simulink model "phdMain"  (R2023b)
settings: Solver=ode4  StartTime=0.0  StopTime=t.Data(end)  FixedStep=1e-3  RelTol=1e-3
undefined symbols (not defined in the file): A_bar, AEFF, B_E, C_bar, C_T, Cd_neg, Cd_pos, DiscIntNeverNeededParam, Gamma, H, k, K, L_gain, L_STROKE, M, m3PsToLpm, P_return_Pa, P_supply_Pa, PA_Pa, PaToBar, PB_Pa, Q, R, RHO, Ts, V01, V02, V_DEAD, v_mPs, W, xc_dot, xc_m
libraries: simulink x1
(part 1 of 3)
settings Model: PauseTimes=22  Creator=snr  LastModifiedBy=snr
settings DataIOCC: OutputOption=AdditionalOutputTimes  OutputTimes=1
settings OptimizationCC: BlockReduction=off  ConditionallyExecuteInputs=off

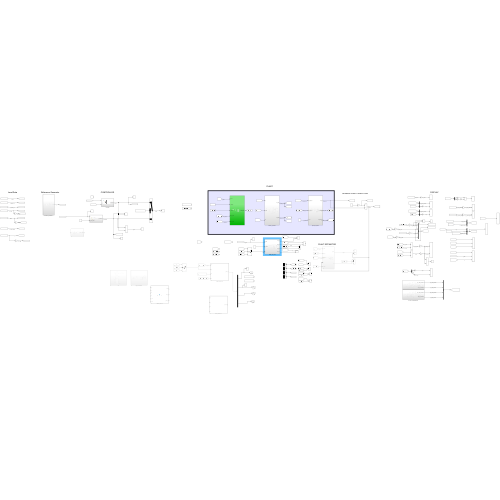
[thumbnail: Simulink's stored preview of the top-level diagram]
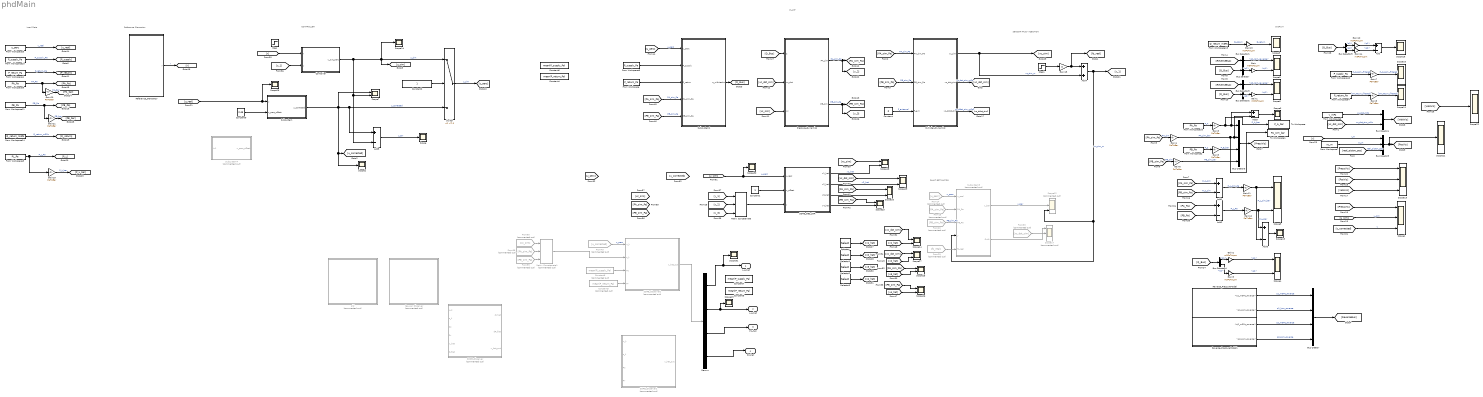
== system phdMain ==
  note: Load Data
  note: PLANT
  note: CONTROLLER
  note: DISPLAY
  note: Reference Generator
  note: SENSOR FAULT INJECTION
  note: FAULT ESTIMATOR
  Add{,1..3,5..6} (6 alike) : Sum  Inputs=+-
  Add4 : Sum
  Bus Selector : BusSelector  OutputSignals=q1
  Bus Selector1 : BusSelector  OutputSignals=q1_lpm_reverse
  Bus Selector2 : BusSelector  OutputSignals=q2
  Bus Selector3 : BusSelector  OutputSignals=q2_lpm_reverse
  Bus Selector4 : BusSelector  OutputSignals=q1,q2
  Bus Selector5 : BusSelector  OutputSignals=q1,q2
  Bus Creator : BusCreator  Inputs=4
  Bus Creator3 : BusCreator  Inputs=4
  Bus Creator4 : BusCreator  Inputs=2
  Bus Creator5 : BusCreator  Inputs=3
  Constant : Constant  Value=0
  Constant1 : Constant
  Constant2 : Constant  OutDataTypeStr=boolean
  Constant3 : Constant  Commented=on  Value=mean(P_return_Pa)
  Constant4 : Constant  Value=mean(P_return_Pa)
  Constant5 : Constant  Value=mean(P_return_Pa)
  Constant6 : Constant  Value=mean(P_supply_Pa)
  Constant7 : Constant  Value=mean(P_supply_Pa)
  Constant8 : Constant  Commented=on  Value=mean(P_supply_Pa)
  Constant9 : Constant  Value=2.45
  Controller : Subsystem
  Cylinder_Dynamics : Subsystem
  Demux : Demux
  From Workspace : FromWorkspace  VariableName=P_return_Pa
  From Workspace1 : FromWorkspace  VariableName=P_return_Pa
  From Workspace10 : FromWorkspace  VariableName=P_supply_Pa
  From Workspace11 : FromWorkspace  VariableName=PB_Pa
  From Workspace12 : FromWorkspace  VariableName=P_supply_Pa
  From Workspace14 : FromWorkspace  VariableName=Q_return_m3Ps
  From Workspace15 : FromWorkspace  VariableName=Q_return_m3Ps
  From Workspace2 : FromWorkspace  VariableName=PB_Pa
  From Workspace20 : FromWorkspace  VariableName=PA_Pa
  From Workspace3 : FromWorkspace  VariableName=u_perc
  From Workspace4 : FromWorkspace  VariableName=P_return_Pa
  From Workspace5 : FromWorkspace  VariableName=PL_Pa
  From Workspace6 : FromWorkspace  VariableName=v_mPs
  From Workspace7 : FromWorkspace  VariableName=xc_m
  From Workspace8 : FromWorkspace  VariableName=P_supply_Pa
  From Workspace9 : FromWorkspace  VariableName=PA_Pa
  From14 : From  Commented=on  GotoTag=u_perc
  From15 : From  Commented=on  GotoTag=PA_sim_Pa
  From20 : From  Commented=on  GotoTag=PB_sim_Pa
  From29 : From  Commented=on  GotoTag=fs_real
  From33 : From  Commented=on  GotoTag=xc_dot_sim
  From43 : From  Commented=on  GotoTag=u_corrected
  From58 : From  Commented=on  GotoTag=PA_sim_Pa
  From59 : From  Commented=on  GotoTag=PB_sim_Pa
  From60 : From  Commented=on  GotoTag=xc_sim
  Gain{,1..2,9..10,13..14} (7 alike) : Gain  Gain=m3PsToLpm
  Gain{3..8,11..12,19..21} (11 alike) : Gain  Gain=PaToBar
  Gain15 : Gain  Gain=0
  Matrix Concatenate : Concatenate  NumInputs=3  Mode=Multidimensional array
  Matrix Concatenate1 : Concatenate  Commented=on  NumInputs=3  Mode=Multidimensional array
  Nguyen Observer : Subsystem  Commented=on
  Pressure_Dynamics : Subsystem
  Reference_Generator : Subsystem
  Reverse_PressureModel : Subsystem
  Reverse_PressureModel1 : Subsystem
  SDRE_OBS_SNR : Subsystem
  SDRE_Observer : MATLAB Function  Commented=on  InitFcn=% x_hat Integrator IC x0_obs = [0; 0; 0; 0]; % 4×1 % P Integrator IC P0 = diag([1e-5, 1e-3, 2e3, 2e3]); % 4×4 P0_flat = P0(:); % 16×1 ← bu kullanılacak  TreatAsAtomicUnit=on
  SDRE_Observer1 : MATLAB Function  Commented=on  TreatAsAtomicUnit=on
  SDRE_Observer2 : MATLAB Function  Commented=on  TreatAsAtomicUnit=on
  Scope{,2..3,8,10..11,14..16,19,21..22,28,30..31} (15 alike) : Scope
  Scope1 : Scope  NumInputPorts=3
  Scope12 : Scope  Commented=on  NumInputPorts=3
  Scope13 : Scope  NumInputPorts=3
  Scope17 : Scope  Commented=on  NumInputPorts=3
  Scope{4..7,9,18,20,23..27,29} (13 alike) : Scope  NumInputPorts=2
  Selector{,1..3} (4 alike) : Selector  InputPortWidth=4  IndexOptions=Index vector (dialog)  Indices=1  OutputSizes=1
  Step : Step  After=10e-3  SampleTime=0
  Step1 : Step  After=5e-3  SampleTime=0
  Subsystem : Subsystem
  Subsystem1 : Subsystem
  Subsystem3 : Subsystem  Commented=on
  Subsystem4 : Subsystem  Commented=on
  Switch : Switch  Criteria=u2 ~= 0  SaturateOnIntegerOverflow=off  InputSameDT=off
  To Workspace : ToWorkspace  VariableName=P_A_bar  SaveFormat=Timeseries  SampleTime=-1
  To Workspace1 : ToWorkspace  VariableName=PA_sim_bar  SaveFormat=Timeseries  SampleTime=-1
  old : Subsystem  Commented=on
  x_c_hat : Outport
  v_c_hat : Outport  Port=2
  P1_hat : Outport  Port=3
  P2_hat : Outport  Port=4
  wires:
  Constant/1 -> Cylinder_Dynamics/3(F_ext)  "F_external"
  Cylinder_Dynamics/2(xc_dot_sim) -> [xc_dot_sim]  "xc_dot_sim_mPs"
  From Workspace7/1 -> Bus Creator5/2  "xc_m"
  [real_piston_pos] -> Bus Creator5/3  "real_piston_pos"
  [xc_dot_sim] -> Bus Creator4/2  "xc_dot_sim_mPs"
  From Workspace6/1 -> Bus Creator4/1  "xc_dot_mPs"
  Pressure_Dynamics/1(PA_sim) -> [y_2], [PA_sim_Pa]  "PA_sim_Pa"
  [PA_sim_Pa] -> Cylinder_Dynamics/1(PA_sim_Pa)  "PA_sim_Pa"
  Pressure_Dynamics/2(PB_sim) -> [y_3], [PB_sim_Pa]  "PB_sim_Pa"
  [PB_sim_Pa] -> Cylinder_Dynamics/2(PB_sim_Pa)  "PB_sim_Pa"
  From Workspace20/1 -> Gain3/1  "P_A"
  [PA_sim_Pa] -> Gain4/1  "PA_sim"
  [PB_sim_Pa] -> Gain6/1  "PB_sim"
  From Workspace2/1 -> Gain5/1  "P_2"
  [Q_Bus] -> Bus Selector/1
  [ReverseBus] -> Bus Selector1/1
  Bus Selector/1 -> Gain/1  "<q1>"
  Bus Selector1/1 -> Scope5/1  "<q1_lpm_reverse>"
  Gain/1 -> Scope5/2  "<q1>"
  Gain1/1 -> Scope6/2  "<q2>"
  Bus Selector3/1 -> Scope6/1  "<q2_lpm_reverse>"
  Bus Selector2/1 -> Gain1/1  "<q2>"
  [ReverseBus] -> Bus Selector3/1
  [Q_Bus] -> Bus Selector2/1
  [xc_sim] -> Pressure_Dynamics/3(xc)
  [xc_dot_sim] -> Pressure_Dynamics/2(xc_dot)
  [PA_sim_Pa] -> Add1/1  "P_1_sim"
  [PB_sim_Pa] -> Add1/2  "P_2_sim"
  Switch/1 -> [u_perc]  "u_sim"
  Add1/1 -> Gain11/1  "P_L_sim_Pa"
  Add2/1 -> Gain12/1  "P_L_Pa"
  Gain3/1 -> To Workspace/1, Add3/1, Bus Creator3/1  "P_A_bar"
  Gain4/1 -> To Workspace1/1, Add3/2, Bus Creator3/2  "PA_sim_bar"
  Gain6/1 -> Bus Creator3/4  "PB_sim_bar"
  Gain5/1 -> Bus Creator3/3  "P_B_bar"
  From Workspace12/1 -> Gain7/1  "P_supply_filtered"
  Gain7/1 -> Scope10/1  "P_supply_filtered"
  Gain8/1 -> Scope11/1  "[t,P_return_filtered]"
  From Workspace4/1 -> Gain8/1  "[t,P_return_filtered]"
  Bus Creator3/1 -> [PressVis]
  [PressVis] -> Scope13/1
  Bus Creator4/1 -> [VeloVis]
  Bus Creator5/1 -> Scope21/1, [PosVis]
  [PressVis] -> Scope1/1
  Gain11/1 -> Add6/2, Scope9/1  "P_L_sim_bar"
  Gain12/1 -> Add6/1, Scope9/2  "P_L_bar"
  Add3/1 -> Scope3/1
  Bus Selector4/1 -> Gain2/1  "<q1>"
  [Q_Bus] -> Bus Selector4/1
  Gain2/1 -> Scope4/1  "<q1>"
  Bus Selector4/2 -> Gain9/1  "<q2>"
  Gain9/1 -> Scope4/2  "<q2>"
  From Workspace15/1 -> Gain13/1  "Q_return"
  Gain13/1 -> Scope8/1  "Q_return"
  [u_corrected] -> Scope1/3  "u"
  Gain10/1 -> Add/1  "<q1>"
  Bus Selector5/1 -> Gain10/1  "<q1>"
  [Q_Bus] -> Bus Selector5/1
  Bus Selector5/2 -> Gain14/1  "<q2>"
  Gain14/1 -> Add/2  "<q2>"
  Add/1 -> Scope16/1
  Constant2/1 -> Switch/2
  Controller/1(u_out_perc) -> Scope7/2, Add5/2, Switch/1, [u_sim], Scope14/1  "u_sim"
  Add4/1 -> [y_1], Scope12/3, Subsystem3/4(y)  "xc_sim_m"
  [u_real] -> Scope28/1, Subsystem/1(u)
  Subsystem/1(u_corrected) -> Scope7/1, [u_corrected], Scope2/1, Add5/1, Switch/3  "u_corrected"
  From Workspace3/1 -> [u_real]  "u_real"
  Reverse_PressureModel/2(<q1_lpm_reverse>) -> Bus Creator/2  "q1_lpm_reverse"
  Bus Creator/1 -> [ReverseBus]
  Reverse_PressureModel/1(<q1_m3Ps_reverse>) -> Bus Creator/1  "q1_m3Ps_reverse"
  Reverse_PressureModel1/1(<q2_m3Ps_reverse>) -> Bus Creator/3  "q2_m3Ps_reverse"
  Reverse_PressureModel1/2(<q2_lpm_reverse>) -> Bus Creator/4  "q2_lpm_reverse"
  From Workspace10/1 -> [P_supply]  "P_supply_Pa"
  From Workspace1/1 -> [P_return]  "P_return_Pa"
  From Workspace9/1 -> Gain20/1, [PA_Pa]  "PA_Pa"
  From Workspace11/1 -> Gain21/1, [PB_Pa]  "PB_Pa"
  Cylinder_Dynamics/3(xc_ddot_sim) -> [xc_ddot_sim]  "xc_ddot_sim_mPs2"
  Reference_Generator/1(r) -> [r]  "r"
  From Workspace14/1 -> [Q_return]  "Q_return_m3Ps"
  [PA_Pa] -> Add2/1
  [PB_Pa] -> Add2/2
  From Workspace5/1 -> [P_L], Gain19/1  "P_L_Pa"
  Gain19/1 -> [P_L_bar]  "P_L_bar"
  Gain20/1 -> [PA_bar]  "PA_bar"
  Gain21/1 -> [PB_bar]  "PB_bar"
  Add5/1 -> Scope/1  "u_err"
  Add6/1 -> Scope15/1
  [Q_Bus] -> Pressure_Dynamics/1(q)
  [u_perc] -> Subsystem1/1(u_perc)  "u_perc"
  From Workspace/1 -> Subsystem1/3(P_return)
  [PA_sim_Pa] -> Subsystem1/4(PA_sim_Pa)  "PA_sim_Pa"
  [PB_sim_Pa] -> Subsystem1/5(PB_sim_Pa)  "PB_sim_Pa"
  [VeloVis] -> Scope13/3
  [PosVis] -> Scope13/2
  Subsystem1/1(q_withLeaks) -> [Q_Bus]
  [r] -> Controller/1(r)
  From Workspace8/1 -> Subsystem1/2(P_supply)
  [u_sim] -> Scope1/2  "u_sim"
  [r] -> Bus Creator5/1  "r_m"
  [VeloVis] -> Scope22/1
  From14/1 -> Subsystem3/1(u_real)  "u_perc"
  From15/1 -> Subsystem3/2(PA_Pa)
  From20/1 -> Subsystem3/3(PB_Pa)  "PB_sim_Pa"
  Subsystem3/1(x_bar) -> Scope12/2  "x_bar"
  Cylinder_Dynamics/1(xc_sim) -> Add4/2, [xc_sim]  "xc_sim_m"
  Step1/1 -> Gain15/1
  Gain15/1 -> [fs_real], Add4/1
  From29/1 -> Subsystem3/5(fs_real)
  From33/1 -> Scope17/2
  Subsystem3/2(Out1) -> Scope17/1
  [u_sim] -> Scope30/1, SDRE_OBS_SNR/1(u_real)  "u_perc"
  [y_1] -> Controller/2(y)
  [y_2] -> Matrix Concatenate/2
  [y_1] -> Matrix Concatenate/1
  [y_3] -> Matrix Concatenate/3
  SDRE_OBS_SNR/1(x1_hat) -> Scope18/2  "x1_hat"
  [xc_sim] -> Scope18/1
  SDRE_OBS_SNR/2(x2_hat) -> Scope29/2  "x2_hat"
  [xc_dot_sim] -> Scope29/1
  SDRE_OBS_SNR/3(x3_hat) -> Scope20/2
  [PA_sim_Pa] -> Scope20/1
  SDRE_OBS_SNR/4(x4_hat) -> Scope23/2
  [PB_sim_Pa] -> Scope23/1
  Selector2/1 -> [x3_hat]
  Selector/1 -> [x1_hat]
  Selector1/1 -> [x2_hat]
  Selector3/1 -> [x4_hat]
  [x1_hat] -> Scope24/2
  [xc_dot_sim] -> Scope24/1
  [PA_sim_Pa] -> Scope25/1
  [x3_hat] -> Scope25/2
  [x4_hat] -> Scope26/2
  [PB_sim_Pa] -> Scope26/1
  [xc_dot_sim] -> Scope27/1
  [x2_hat] -> Scope27/2
  Constant1/1 -> SDRE_OBS_SNR/2(u_offset)
  Matrix Concatenate/1 -> SDRE_OBS_SNR/3(y)
  Demux/4 -> P2_hat/1
  Matrix Concatenate1/1 -> SDRE_Observer2/2(z_k)
  Demux/3 -> P1_hat/1
  From59/1 -> Matrix Concatenate1/3
  From60/1 -> Matrix Concatenate1/1
  From58/1 -> Matrix Concatenate1/2
  From43/1 -> SDRE_Observer2/1(u_k)  "u_perc"
  Constant8/1 -> SDRE_Observer2/3(Ps)
  Constant9/1 -> Subsystem/2(u_perc_offset)
  Demux/2 -> Scope19/1, v_c_hat/1
  Constant3/1 -> SDRE_Observer2/4(Pr)
  SDRE_Observer2/1(x_hat_out) -> Demux/1
  Demux/1 -> Scope31/1, x_c_hat/1

== system phdMain/Controller ==
  note: Offset - Yapmaya İhtiyaç yok
  note: Integral Gain
  note: Proportional Gain
  r : Inport  OutDataTypeStr=double
  y : Inport  Port=2  OutDataTypeStr=double
  Add : Sum
  Add1 : Sum  Inputs=+-
  Add3 : Sum
  Constant : Constant  Value=45
  Constant1 : Constant  Value=5
  Constant2 : Constant  Value=0  OutDataTypeStr=double
  Gain1 : Gain  Gain=1000
  Integrator : Integrator
  Product : Product
  Product1 : Product
  Saturation : Saturate  UpperLimit=100  LowerLimit=-100
  u_out_perc : Outport  OutDataTypeStr=double
  wires:
  Constant/1 -> Product/1
  Constant1/1 -> Product1/1
  Add1/1 -> Product1/2, Product/2  "e"
  Product/1 -> Integrator/1
  Integrator/1 -> Add/2
  r/1 -> Add1/1  "r"
  Add/1 -> Gain1/1
  y/1 -> Add1/2
  Add3/1 -> Saturation/1
  Gain1/1 -> Add3/2
  Saturation/1 -> u_out_perc/1
  Product1/1 -> Add/1
  Constant2/1 -> Add3/1

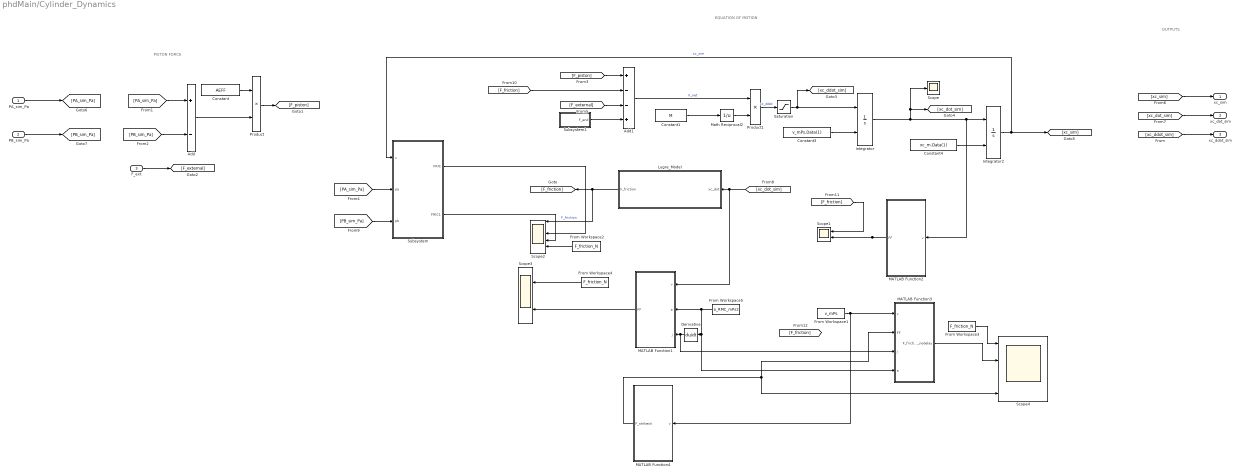
== system phdMain/Cylinder_Dynamics ==
  note: PISTON FORCE
  note: EQUATION OF MOTION
  note: OUTPUTS
  PA_sim_Pa : Inport  OutDataTypeStr=double
  PB_sim_Pa : Inport  Port=2  OutDataTypeStr=double
  F_ext : Inport  Port=3  OutDataTypeStr=double
  Add : Sum  Inputs=+-
  Add1 : Sum  Inputs=+--+
  Constant : Constant  Value=AEFF  OutDataTypeStr=double
  Constant1 : Constant  Value=M  OutDataTypeStr=double
  Constant3 : Constant  Value=v_mPs.Data(1)
  Constant4 : Constant  Value=xc_m.Data(1)
  Derivative : Derivative
  From Workspace1 : FromWorkspace  VariableName=v_mPs
  From Workspace2 : FromWorkspace  VariableName=F_friction_N
  From Workspace3 : FromWorkspace  VariableName=F_friction_N
  From Workspace4 : FromWorkspace  VariableName=F_friction_N
  From Workspace5 : FromWorkspace  VariableName=a_RMC_mPs2
  Integrator : Integrator  InitialConditionSource=external  InitialCondition=xc_dot(1)  UpperSaturationLimit=4  LowerSaturationLimit=-4
  Integrator2 : Integrator  InitialConditionSource=external  InitialCondition=xc_dot(1)  LimitOutput=on  UpperSaturationLimit=0.09580  LowerSaturationLimit=-0.09580
  Lugre_Model : Subsystem
  MATLAB Function1 : MATLAB Function  TreatAsAtomicUnit=on
  MATLAB Function2 : MATLAB Function  TreatAsAtomicUnit=on
  MATLAB Function3 : MATLAB Function  TreatAsAtomicUnit=on
  MATLAB Function4 : MATLAB Function  TreatAsAtomicUnit=on
  Math Reciprocal2 : Math  Operator=reciprocal  SignedPower=on
  Product : Product
  Product1 : Product
  Saturation : Saturate  UpperLimit=100  LowerLimit=-100
  Scope : Scope
  Scope1 : Scope  NumInputPorts=2
  Scope2 : Scope  NumInputPorts=6
  Scope3 : Scope  NumInputPorts=2
  Scope4 : Scope  NumInputPorts=4
  Subsystem : Subsystem
  Subsystem1 : Subsystem
  xc_sim : Outport  OutDataTypeStr=double
  xc_dot_sim : Outport  Port=2  OutDataTypeStr=double
  xc_ddot_sim : Outport  Port=3  OutDataTypeStr=double
  wires:
  [PB_sim_Pa] -> Add/2
  [PA_sim_Pa] -> Add/1
  Add/1 -> Product/2
  Constant/1 -> Product/1
  Math Reciprocal2/1 -> Product1/2
  Product1/1 -> Saturation/1  "xc_ddot"
  Product/1 -> [F_piston]
  F_ext/1 -> [F_external]
  Add1/1 -> Product1/1  "F_net"
  Constant3/1 -> Integrator/2
  Integrator/1 -> MATLAB Function2/1(v), Integrator2/1, Scope/1, [xc_dot_sim]
  Constant4/1 -> Integrator2/2
  Integrator2/1 -> Subsystem/1(x), [xc_sim]  "xc_sim"
  [xc_sim] -> xc_sim/1
  [xc_dot_sim] -> xc_dot_sim/1
  [xc_dot_sim] -> MATLAB Function1/1(v), Lugre_Model/1(xc_dot)
  [xc_ddot_sim] -> xc_ddot_sim/1
  Saturation/1 -> [xc_ddot_sim], Integrator/1
  [F_external] -> Add1/3
  [F_piston] -> Add1/1
  Lugre_Model/1(F_friction) -> Scope2/1, [F_friction]  "F_friction"
  From Workspace2/1 -> Scope2/5
  Subsystem1/1(F_end) -> Add1/4
  PA_sim_Pa/1 -> [PA_sim_Pa]
  PB_sim_Pa/1 -> [PB_sim_Pa]
  [PA_sim_Pa] -> Subsystem/2(pa)
  [PB_sim_Pa] -> Subsystem/3(pb)
  Constant1/1 -> Math Reciprocal2/1
  Subsystem/2(FRIC1) -> Scope2/4
  Subsystem/1(FRIC) -> Scope2/3
  Derivative/1 -> MATLAB Function3/3(j), MATLAB Function1/3(j)
  From Workspace4/1 -> Scope3/1
  MATLAB Function1/1(FF) -> Scope3/2
  From Workspace5/1 -> MATLAB Function3/4(a), Derivative/1, MATLAB Function1/2(a)
  MATLAB Function2/1(FF) -> Scope1/2
  [F_friction] -> Scope1/1
  From Workspace1/1 -> MATLAB Function4/1(v), MATLAB Function3/1(v)
  MATLAB Function3/1(F_friction_nodelay) -> Scope4/2
  From Workspace3/1 -> Scope4/1
  MATLAB Function4/1(F_stribeck) -> MATLAB Function3/2(FF), Scope4/4
  [F_friction] -> Add1/2

== system phdMain/Nguyen Observer ==
  note: [1000; 1000; 1e-6; 1e-6]
  Add4 : Sum  Commented=on  Inputs=+-
  From Workspace13 : FromWorkspace  Commented=on  VariableName=P_return_Pa
  From Workspace16 : FromWorkspace  Commented=on  VariableName=P_supply_Pa
  From Workspace17 : FromWorkspace  Commented=on  VariableName=PB_Pa
  From Workspace18 : FromWorkspace  Commented=on  VariableName=PA_Pa
  From14 : From  Commented=on  GotoTag=u_perc
  From15 : From  Commented=on  GotoTag=xc_sim
  From20 : From  Commented=on  GotoTag=xc_dot_sim
  From29 : From  Commented=on  GotoTag=x1_hat
  From32 : From  Commented=on  GotoTag=xc_sim
  From33 : From  Commented=on  GotoTag=x2_hat
  From36 : From  Commented=on  GotoTag=fs_hat
  From37 : From  Commented=on  GotoTag=PA_sim_Pa
  From38 : From  Commented=on  GotoTag=x3_hat
  From40 : From  Commented=on  GotoTag=xc_dot_sim
  Gain15 : Gain  Commented=on  Gain=[1000; 1000; 1e-6; 1e-6]
  Goto21 : Goto  Commented=on  GotoTag=x1_hat
  Goto22 : Goto  Commented=on  GotoTag=x3_hat
  Goto26 : Goto  Commented=on  GotoTag=fs_hat
  Goto27 : Goto  Commented=on  GotoTag=x4_hat
  Goto28 : Goto  Commented=on  GotoTag=x2_hat
  Matrix Concatenate : Concatenate  Commented=on  NumInputs=4  Mode=Multidimensional array
  Nguyen_Observer : Subsystem  Commented=on
  Scope12 : Scope  Commented=on  NumInputPorts=2
  Scope17 : Scope  Commented=on  NumInputPorts=2
  Scope18 : Scope  Commented=on
  Scope19 : Scope  Commented=on
  Scope20 : Scope  Commented=on  NumInputPorts=2
  Selector : Selector  Commented=on  InputPortWidth=5  IndexOptions=Index vector (dialog)  Indices=1  OutputSizes=1
  Selector1 : Selector  Commented=on  InputPortWidth=5  IndexOptions=Index vector (dialog)  Indices=2  OutputSizes=1
  Selector2 : Selector  Commented=on  InputPortWidth=5  IndexOptions=Index vector (dialog)  Indices=3  OutputSizes=1
  Selector3 : Selector  Commented=on  InputPortWidth=5  IndexOptions=Index vector (dialog)  Indices=4  OutputSizes=1
  Selector4 : Selector  Commented=on  InputPortWidth=5  IndexOptions=Index vector (dialog)  Indices=5  OutputSizes=1
  Zero-Order Hold3 : ZeroOrderHold  Commented=on  SampleTime=Ts
  wires:
  From Workspace13/1 -> Nguyen_Observer/3(P_return)
  Add4/1 -> Scope19/1
  From Workspace17/1 -> Matrix Concatenate/4
  Selector4/1 -> Goto26/1
  From14/1 -> Nguyen_Observer/1(u_perc)  "u_perc"
  Selector2/1 -> Goto22/1
  Matrix Concatenate/1 -> Zero-Order Hold3/1
  From38/1 -> Scope20/2
  From Workspace16/1 -> Nguyen_Observer/2(P_supply)
  From32/1 -> Add4/1, Scope12/1
  Zero-Order Hold3/1 -> Gain15/1
  From36/1 -> Scope18/1
  From40/1 -> Scope17/1
  Gain15/1 -> Nguyen_Observer/4(y)
  From20/1 -> Matrix Concatenate/2
  From15/1 -> Matrix Concatenate/1
  Selector/1 -> Goto21/1
  Selector3/1 -> Goto27/1
  From37/1 -> Scope20/1  "PA_sim_Pa"
  Selector1/1 -> Goto28/1
  From Workspace18/1 -> Matrix Concatenate/3
  Nguyen_Observer/1(xbar_hat_safe) -> Selector4/1, Selector3/1, Selector2/1, Selector1/1, Selector/1
  From33/1 -> Scope17/2
  From29/1 -> Add4/2, Scope12/2

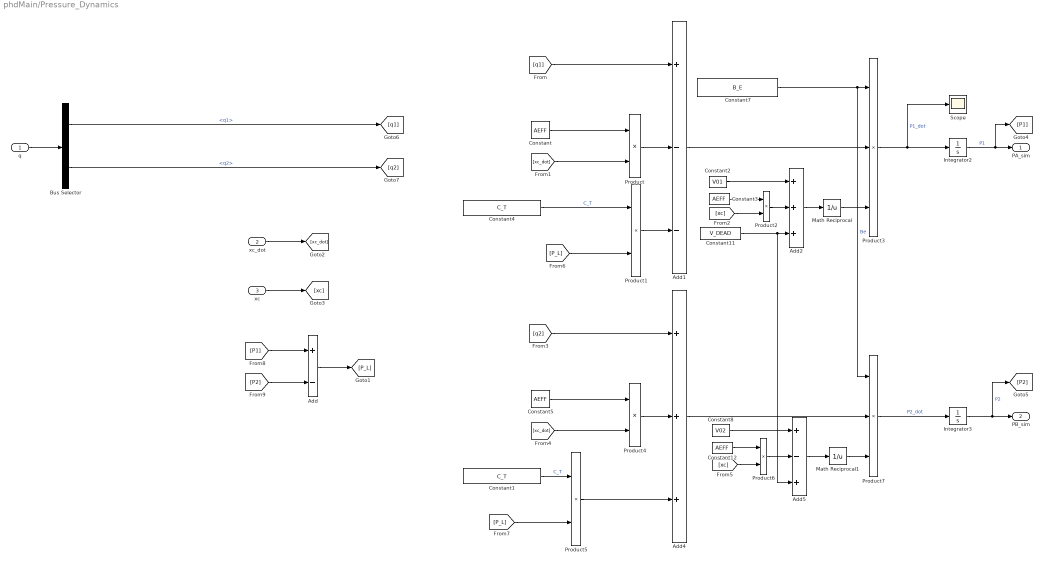
== system phdMain/Pressure_Dynamics ==
  q : Inport  OutDataTypeStr=double
  xc_dot : Inport  Port=2  OutDataTypeStr=double
  xc : Inport  Port=3  OutDataTypeStr=double
  Add : Sum  Inputs=+-
  Add1 : Sum  Inputs=+--
  Add2 : Sum  Inputs=+++
  Add4 : Sum  Inputs=+++
  Add5 : Sum  Inputs=+-+
  Bus Selector : BusSelector  OutputSignals=q1,q2
  Constant{,3,5,12} (4 alike) : Constant  Value=AEFF  OutDataTypeStr=double
  Constant1 : Constant  Value=C_T  OutDataTypeStr=double
  Constant11 : Constant  Value=V_DEAD  OutDataTypeStr=double
  Constant2 : Constant  Value=V01  OutDataTypeStr=double
  Constant4 : Constant  Value=C_T  OutDataTypeStr=double
  Constant7 : Constant  Value=B_E  OutDataTypeStr=double
  Constant8 : Constant  Value=V02  OutDataTypeStr=double
  Integrator2 : Integrator  InitialCondition=PA_Pa.Data(1)  LimitOutput=on  UpperSaturationLimit=200e5  LowerSaturationLimit=4e5
  Integrator3 : Integrator  InitialCondition=PB_Pa.Data(1)  LimitOutput=on  UpperSaturationLimit=200e5  LowerSaturationLimit=4e5
  Math Reciprocal : Math  Operator=reciprocal  SignedPower=on
  Math Reciprocal1 : Math  Operator=reciprocal  SignedPower=on
  Product{,1..2,4..6} (6 alike) : Product
  Product3 : Product  Inputs=3
  Product7 : Product  Inputs=3
  Scope : Scope
  PA_sim : Outport  OutDataTypeStr=double
  PB_sim : Outport  Port=2  OutDataTypeStr=double
  wires:
  q/1 -> Bus Selector/1
  xc_dot/1 -> [xc_dot]
  [xc_dot] -> Product/2
  Constant/1 -> Product/1
  Integrator2/1 -> [P1], PA_sim/1  "P1"
  [P_L] -> Product1/2
  Product/1 -> Add1/2
  [q1] -> Add1/1
  xc/1 -> [xc]
  Constant2/1 -> Add2/1
  Product2/1 -> Add2/2
  [xc] -> Product2/2
  Constant3/1 -> Product2/1
  Add2/1 -> Math Reciprocal/1
  Product3/1 -> Integrator2/1, Scope/1  "P1_dot"
  Math Reciprocal/1 -> Product3/3
  Add1/1 -> Product3/2
  Constant7/1 -> Product7/1, Product3/1  "Be"
  Constant4/1 -> Product1/1  "C_T"
  [xc_dot] -> Product4/2
  Product4/1 -> Add4/2
  Add4/1 -> Product7/2
  Integrator3/1 -> [P2], PB_sim/1  "P2"
  [P_L] -> Product5/2
  Constant5/1 -> Product4/1
  Add5/1 -> Math Reciprocal1/1
  [q2] -> Add4/1
  Math Reciprocal1/1 -> Product7/3
  Product7/1 -> Integrator3/1  "P2_dot"
  [xc] -> Product6/2
  Constant8/1 -> Add5/1
  Constant12/1 -> Product6/1
  Product6/1 -> Add5/2
  Bus Selector/2 -> [q2]  "<q2>"
  Bus Selector/1 -> [q1]  "<q1>"
  [P2] -> Add/2
  [P1] -> Add/1
  Add/1 -> [P_L]
  Constant1/1 -> Product5/1  "C_T"
  Product5/1 -> Add4/3
  Product1/1 -> Add1/3
  Constant11/1 -> Add5/3, Add2/3

== system phdMain/Reference_Generator ==
  Band-Limited White Noise : simulink/Sources/Band-Limited White Noise  Cov=[0.001]  Ts=5  seed=[23341]
  Constant : Constant  Value=0  OutDataTypeStr=uint8
  Constant1 : Constant  Commented=on  Value=30  OutDataTypeStr=double
  Constant2 : Constant  Commented=on  OutDataTypeStr=double
  Constant3 : Constant  Commented=on  Value=0  OutDataTypeStr=double
  Constant4 : Constant  Value=0
  Constant5 : Constant  Value=0
  From Workspace14 : FromWorkspace  VariableName=r_m
  Multiport Switch : MultiPortSwitch  DataPortOrder=Zero-based contiguous  DataPortForDefault=Additional data port  zeroidx=on  OutDataTypeStr=double  SaturateOnIntegerOverflow=off  InputSameDT=off
  Saturation : Saturate  UpperLimit=0.09580  LowerLimit=-0.09580
  Scope : Scope
  Sine Wave : Sin  Amplitude=30e-3  Frequency=pi  SampleTime=0
  Sine_Generator : Subsystem  Commented=on
  r : Outport  OutDataTypeStr=double
  wires:
  From Workspace14/1 -> Multiport Switch/2  "r_m"
  Constant/1 -> Multiport Switch/1
  Constant1/1 -> Sine_Generator/1(Amp_mm)
  Constant2/1 -> Sine_Generator/2(f_Hz)
  Constant3/1 -> Sine_Generator/3(phi_deg)
  Band-Limited White Noise/1 -> Saturation/1
  Saturation/1 -> Multiport Switch/4
  Multiport Switch/1 -> Scope/1, r/1
  Constant4/1 -> Multiport Switch/5
  Constant5/1 -> Multiport Switch/3

== system phdMain/Reverse_PressureModel ==
  Abs : Abs  SaturateOnIntegerOverflow=off
  Add : Sum  Inputs=+-
  Add1 : Sum  Inputs=+++
  Add2 : Sum
  Add3 : Sum  Inputs=+-
  Constant : Constant  Value=AEFF  OutDataTypeStr=double
  Constant1 : Constant  Value=C_T  OutDataTypeStr=double
  Constant2 : Constant  Value=V01  OutDataTypeStr=double
  Constant3 : Constant  Value=AEFF  OutDataTypeStr=double
  Constant4 : Constant  Value=B_E  OutDataTypeStr=double
  Derivative : Derivative
  From Workspace1 : FromWorkspace  VariableName=Q_return_m3Ps
  From Workspace11 : FromWorkspace  VariableName=v_mPs
  From Workspace12 : FromWorkspace  VariableName=xc_m
  From Workspace15 : FromWorkspace  VariableName=PA_Pa
  From Workspace2 : FromWorkspace  VariableName=PB_Pa
  Gain : Gain  Gain=60e3
  Gain1 : Gain  Gain=60e3
  Math Reciprocal : Math  Operator=reciprocal  SignedPower=on
  Product : Product
  Product1 : Product
  Product2 : Product
  Product3 : Product  Inputs=3
  Q_returnleak : Subsystem
  Scope : Scope
  Scope2 : Scope  NumInputPorts=4
  <q1_m3Ps_reverse> : Outport
  <q1_lpm_reverse> : Outport  Port=2
  wires:
  From Workspace12/1 -> [xc]
  Gain/1 -> <q1_lpm_reverse>/1, Abs/1, Scope2/1  "<q1_lpm_reverse>"
  Gain1/1 -> Add/1, Scope2/2  "<Q_return_filtered_lpm>"
  From Workspace1/1 -> Gain1/1  "Q_return_filtered"
  Product2/1 -> Add2/2
  Product3/1 -> Add1/2
  Math Reciprocal/1 -> Product3/1
  Add1/1 -> Scope/1, Gain/1, <q1_m3Ps_reverse>/1  "<q1_m3Ps_reverse>"
  From Workspace15/1 -> Add3/1, Derivative/1  "P_1"
  [xc] -> Product2/2
  Constant2/1 -> Add2/1
  Constant3/1 -> Product2/1
  Abs/1 -> Scope2/3
  Add2/1 -> Product3/3
  Constant4/1 -> Math Reciprocal/1
  From Workspace11/1 -> [xc_dot]
  Product/1 -> Add1/1
  Constant/1 -> Product/1
  [xc_dot] -> Product/2
  Q_returnleak/1(Out1) -> Add/2
  Add/1 -> Scope2/4
  Add3/1 -> Product1/2
  Product1/1 -> Add1/3
  Constant1/1 -> Product1/1
  From Workspace2/1 -> Add3/2  "P_2"
  Derivative/1 -> Product3/2

== system phdMain/Reverse_PressureModel1 ==
  Abs : Abs  SaturateOnIntegerOverflow=off
  Add : Sum  Inputs=+-
  Add1 : Sum  Inputs=-+-
  Add2 : Sum  Inputs=+-
  Add3 : Sum  Inputs=+-
  Constant : Constant  Value=AEFF  OutDataTypeStr=double
  Constant1 : Constant  Value=C_T  OutDataTypeStr=double
  Constant2 : Constant  Value=V02  OutDataTypeStr=double
  Constant4 : Constant  Value=B_E  OutDataTypeStr=double
  Constant5 : Constant  Value=AEFF  OutDataTypeStr=double
  Derivative : Derivative
  From Workspace1 : FromWorkspace  VariableName=Q_return_m3Ps
  From Workspace3 : FromWorkspace  VariableName=v_mPs
  From Workspace4 : FromWorkspace  VariableName=PA_Pa
  From Workspace5 : FromWorkspace  VariableName=xc_m
  From Workspace6 : FromWorkspace  VariableName=PB_Pa
  Gain : Gain  Gain=60e3
  Gain1 : Gain  Gain=60e3
  Math Reciprocal : Math  Operator=reciprocal  SignedPower=on
  Product : Product
  Product1 : Product
  Product2 : Product
  Product3 : Product  Inputs=3
  Q_returnleak : Subsystem
  Scope : Scope
  Scope2 : Scope  NumInputPorts=4
  <q2_m3Ps_reverse> : Outport
  <q2_lpm_reverse> : Outport  Port=2
  wires:
  Derivative/1 -> Product3/2
  From Workspace6/1 -> Add3/2  "P_2"
  Constant1/1 -> Product1/1
  Product1/1 -> Add1/3
  Add3/1 -> Product1/2
  Add/1 -> Scope2/4
  Q_returnleak/1(Out1) -> Add/2
  [xc_dot] -> Product/2
  Constant/1 -> Product/1
  Product/1 -> Add1/1
  From Workspace3/1 -> [xc_dot]
  Constant4/1 -> Math Reciprocal/1
  Add2/1 -> Product3/3
  Abs/1 -> Scope2/3
  Constant5/1 -> Product2/1
  Constant2/1 -> Add2/1
  [xc] -> Product2/2
  From Workspace4/1 -> Derivative/1, Add3/1  "P_1"
  Add1/1 -> <q2_m3Ps_reverse>/1, Gain/1, Scope/1  "<q2_m3Ps_reverse>"
  Math Reciprocal/1 -> Product3/1
  Product3/1 -> Add1/2
  Product2/1 -> Add2/2
  From Workspace1/1 -> Gain1/1  "Q_return_filtered"
  Gain1/1 -> Scope2/2, Add/1  "<Q_return_filtered_lpm>"
  Gain/1 -> Scope2/1, Abs/1, <q2_lpm_reverse>/1  "<q2_lpm_reverse>"
  From Workspace5/1 -> [xc]

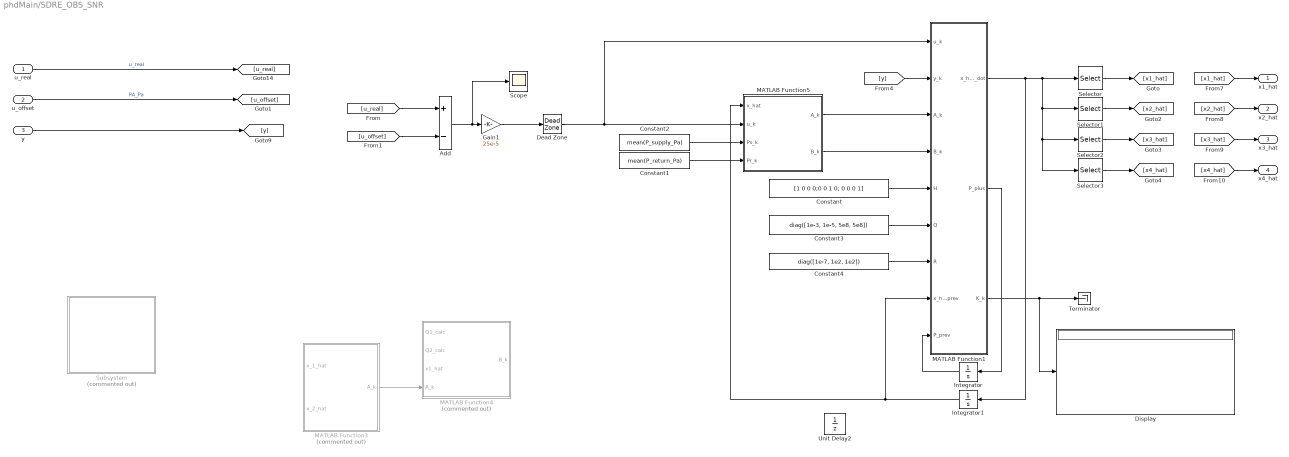
== system phdMain/SDRE_OBS_SNR ==
  u_real : Inport  PortDimensions=[1,1]
  u_offset : Inport  Port=2  Unit=1  PortDimensions=[1,1]
  y : Inport  Port=3  PortDimensions=[3,1]
  Add : Sum  Inputs=+-
  Constant : Constant  Value=[1 0 0 0;0 0 1 0; 0 0 0 1]
  Constant1 : Constant  Value=mean(P_return_Pa)
  Constant2 : Constant  Value=mean(P_supply_Pa)
  Constant3 : Constant  Value=diag([1e-3, 1e-5, 5e8, 5e8])
  Constant4 : Constant  Value=diag([1e-7, 1e2, 1e2])
  Dead Zone : DeadZone  LowerValue=-0.02  UpperValue=0.02
  Display : Display
  Gain1 : Gain  Gain=25e-5
  Integrator : Integrator  InitialCondition=diag([1e-5, 1e-3, 2e3, 2e3])
  Integrator1 : Integrator  InitialCondition=[0; 0; PA_Pa.Data(1); PB_Pa.Data(1)]
  MATLAB Function1 : MATLAB Function  TreatAsAtomicUnit=on
  MATLAB Function3 : MATLAB Function  Commented=on  TreatAsAtomicUnit=on
  MATLAB Function4 : MATLAB Function  Commented=on  TreatAsAtomicUnit=on
  MATLAB Function5 : MATLAB Function  TreatAsAtomicUnit=on
  Scope : Scope
  Selector : Selector  InputPortWidth=4  IndexOptions=Index vector (dialog)  Indices=1  OutputSizes=1
  Selector1 : Selector  InputPortWidth=4  IndexOptions=Index vector (dialog)  Indices=2  OutputSizes=1
  Selector2 : Selector  InputPortWidth=4  IndexOptions=Index vector (dialog)  Indices=3  OutputSizes=1
  Selector3 : Selector  InputPortWidth=4  IndexOptions=Index vector (dialog)  Indices=4  OutputSizes=1
  Subsystem : Subsystem  Commented=on
  Terminator : Terminator
  Unit Delay2 : UnitDelay  InitialCondition=[0; 0; PA_Pa.Data(1); PB_Pa.Data(1)]  SampleTime=1e-3  HasFrameUpgradeWarning=on
  x1_hat : Outport
  x2_hat : Outport  Port=2
  x3_hat : Outport  Port=3
  x4_hat : Outport  Port=4
  wires:
  u_real/1 -> [u_real]  "u_real"
  u_offset/1 -> [u_offset]  "PA_Pa"
  [u_real] -> Add/1
  [u_offset] -> Add/2
  Add/1 -> Scope/1, Gain1/1
  MATLAB Function5/1(A_k) -> MATLAB Function1/3(A_k)
  y/1 -> [y]
  MATLAB Function1/1(x_hat_dot) -> Integrator1/1, Selector3/1, Selector2/1, Selector1/1, Selector/1
  Selector/1 -> [x1_hat]
  Selector1/1 -> [x2_hat]
  Selector2/1 -> [x3_hat]
  Selector3/1 -> [x4_hat]
  [x1_hat] -> x1_hat/1
  [x2_hat] -> x2_hat/1
  [x3_hat] -> x3_hat/1
  [x4_hat] -> x4_hat/1
  MATLAB Function5/2(B_k) -> MATLAB Function1/4(B_k)
  Dead Zone/1 -> MATLAB Function1/1(u_k), MATLAB Function5/2(u_k)
  MATLAB Function3/1(A_k) -> MATLAB Function4/4(A_k)
  MATLAB Function1/2(P_plus) -> Integrator/1
  Integrator/1 -> MATLAB Function1/9(P_prev)
  MATLAB Function1/3(K_k) -> Display/1, Terminator/1
  Constant/1 -> MATLAB Function1/5(H)
  Constant3/1 -> MATLAB Function1/6(Q)
  Constant4/1 -> MATLAB Function1/7(R)
  [y] -> MATLAB Function1/2(y_k)
  Integrator1/1 -> MATLAB Function1/8(x_hat_prev), MATLAB Function5/1(x_hat)
  Gain1/1 -> Dead Zone/1
  Constant1/1 -> MATLAB Function5/4(Pr_k)
  Constant2/1 -> MATLAB Function5/3(Ps_k)

== system phdMain/Subsystem ==
  u : Inport  OutDataTypeStr=double
  u_perc_offset : Inport  Port=2  OutDataTypeStr=double
  Add : Sum  Inputs=+-
  u_corrected : Outport
  wires:
  u/1 -> Add/1
  u_perc_offset/1 -> Add/2
  Add/1 -> u_corrected/1

== system phdMain/Subsystem1 ==
  note: Deadband
  u_perc : Inport  OutDataTypeStr=double
  P_supply : Inport  Port=2  OutDataTypeStr=double
  P_return : Inport  Port=3  OutDataTypeStr=double
  PA_sim_Pa : Inport  Port=4  OutDataTypeStr=double
  PB_sim_Pa : Inport  Port=5  OutDataTypeStr=double
  Bus Creator4 : BusCreator  Inputs=2
  Constant1 : Constant  Value=0.01
  Constant2 : Constant  Value=25e-3
  Constant4 : Constant  Value=k
  Constant7 : Constant  Value=K
  Dead Zone : DeadZone  LowerValue=-0.02  UpperValue=0.02
  From Workspace2 : FromWorkspace  VariableName=Q_return_m3Ps
  Gain1 : Gain  Gain=m3PsToLpm
  Gain2 : Gain  Gain=m3PsToLpm
  MATLAB Function : MATLAB Function  TreatAsAtomicUnit=on
  Product : Product  Inputs=3
  Scope : Scope
  Scope1 : Scope  NumInputPorts=2
  Scope2 : Scope  NumInputPorts=2
  Valve Dynamics : TransferFcn  Numerator=[2.0884e+06]  Denominator=[1 2*1*1.4451e+03 2.0884e+06]
  q_withLeaks : Outport  OutDataTypeStr=double
  wires:
  PA_sim_Pa/1 -> [P_A]
  P_supply/1 -> [P_supply]
  P_return/1 -> [P_return]
  PB_sim_Pa/1 -> [P_B]
  u_perc/1 -> [u_perc]
  [P_supply] -> MATLAB Function/2(Ps)
  [P_return] -> MATLAB Function/3(Pr)
  [P_A] -> MATLAB Function/4(P1)
  [P_B] -> MATLAB Function/5(P2)
  Bus Creator4/1 -> q_withLeaks/1
  MATLAB Function/1(Q1) -> Bus Creator4/1  "q1"
  MATLAB Function/2(Q2) -> Bus Creator4/2  "q2"
  Constant2/1 -> Product/1
  Product/1 -> Scope/1, MATLAB Function/1(x)  "i"
  Constant1/1 -> Product/2
  Gain1/1 -> Scope1/2  "Q_return_lpm"
  From Workspace2/1 -> Gain1/1
  MATLAB Function/3(QR) -> Gain2/1
  Gain2/1 -> Scope1/1  "Q_return_calc_lpm"
  [u_perc] -> Scope2/1, Dead Zone/1
  Dead Zone/1 -> Valve Dynamics/1
  Constant4/1 -> MATLAB Function/7(k)
  Constant7/1 -> MATLAB Function/6(K)
  Valve Dynamics/1 -> Scope2/2, Product/3

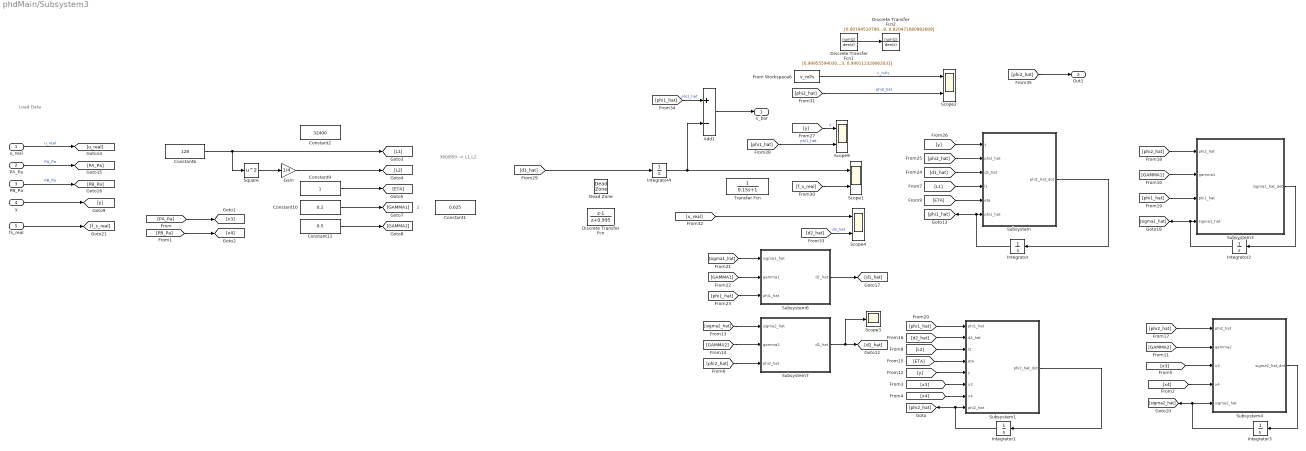
== system phdMain/Subsystem3 ==
  note: 2
  note: 360/850 -> L1,L2
  note: Load Data
  u_real : Inport
  PA_Pa : Inport  Port=2
  PB_Pa : Inport  Port=3
  y : Inport  Port=4
  fs_real : Inport  Port=5
  Add1 : Sum  Inputs=+-
  Constant1 : Constant  Value=0.625
  Constant10 : Constant  Value=0.2
  Constant11 : Constant  Value=0.5
  Constant2 : Constant  Value=32400
  Constant6 : Constant  Value=128
  Constant9 : Constant
  Dead Zone : DeadZone  LowerValue=-0.01  UpperValue=0.01
  Discrete Transfer Fcn : DiscreteTransferFcn  Numerator=[1 -1]  Denominator=[1 0.995]
  Discrete Transfer Fcn1 : DiscreteTransferFcn  Numerator=[0.999555940307616, -1.999111880615232, 0.999555940307616]  Denominator=[1.000000000000000, -1.999111432168433, 0.999112329062031]
  Discrete Transfer Fcn2 : DiscreteTransferFcn  Numerator=[0.001945107908955, 0.003890215817911, 0.001945107908955]  Denominator=[1.000000000000000, -1.812690649346788, 0.820471080982609]
  From Workspace6 : FromWorkspace  VariableName=v_mPs
  Gain : Gain  Gain=1/4
  Integrator{,1..4} (5 alike) : Integrator
  Scope{1..2,4,9} (4 alike) : Scope  NumInputPorts=2
  Scope3 : Scope
  Square : Math  Operator=square
  Subsystem : Subsystem
  Subsystem1 : Subsystem
  Subsystem3 : Subsystem
  Subsystem4 : Subsystem
  Subsystem6 : Subsystem
  Subsystem7 : Subsystem
  Transfer Fcn : TransferFcn  Denominator=[0.15 1]
  x_bar : Outport
  Out1 : Outport  Port=2
  wires:
  [u_real] -> Scope4/1
  Subsystem4/1(sigma2_hat_dot) -> Integrator3/1
  Constant6/1 -> Square/1, [L1]
  [y] -> Subsystem/1(y)
  Constant9/1 -> [ETA]
  [GAMMA2] -> Subsystem7/2(gamma2)
  [GAMMA1] -> Subsystem3/2(gamma1)
  Subsystem/1(phi1_hat_dot) -> Integrator/1
  Gain/1 -> [L2]
  [GAMMA1] -> Subsystem6/2(gamma1)
  [y] -> Subsystem1/5(y)
  Constant10/1 -> [GAMMA1]
  y/1 -> [y]
  [GAMMA2] -> Subsystem4/2(gamma2)
  Subsystem7/1(d2_hat) -> Scope3/1, [d2_hat]
  [L2] -> Subsystem1/3(l2)
  Subsystem6/1(d1_hat) -> [d1_hat]
  [phi1_hat] -> Subsystem3/3(phi1_hat)
  [ETA] -> Subsystem/5(eta)
  [phi1_hat] -> Scope9/2  "phi1_hat"
  Integrator/1 -> [phi1_hat], Subsystem/6(phi1_hat)
  [d2_hat] -> Subsystem1/2(d2_hat)
  Constant11/1 -> [GAMMA2]
  [d2_hat] -> Scope4/2  "d2_hat"
  [phi2_hat] -> Subsystem7/3(phi2_hat)
  [y] -> Scope9/1  "y"
  [phi2_hat] -> Subsystem4/1(phi2_hat)
  [sigma1_hat] -> Subsystem6/1(sigma1_hat)
  [L1] -> Subsystem/4(l1)
  Integrator2/1 -> [sigma1_hat], Subsystem3/4(sigma1_hat)
  [PA_Pa] -> [x3]
  [x3] -> Subsystem1/6(x3)
  PB_Pa/1 -> [PB_Pa]  "PB_Pa"
  u_real/1 -> [u_real]  "u_real"
  Subsystem3/1(sigma1_hat_dot) -> Integrator2/1
  [ETA] -> Subsystem1/4(eta)
  [phi1_hat] -> Subsystem6/3(phi1_hat)
  Integrator3/1 -> Subsystem4/5(sigma2_hat), [sigma2_hat]
  [sigma2_hat] -> Subsystem7/1(sigma2_hat)
  [x3] -> Subsystem4/3(x3)
  [x4] -> Subsystem4/4(x4)
  [d1_hat] -> Subsystem/3(d1_hat)
  From Workspace6/1 -> Scope2/1  "v_mPs"
  [phi1_hat] -> Subsystem1/1(phi1_hat)
  [phi2_hat] -> Subsystem/2(phi2_hat)
  [phi2_hat] -> Subsystem3/1(phi2_hat)
  [x4] -> Subsystem1/7(x4)
  PA_Pa/1 -> [PA_Pa]  "PA_Pa"
  [PB_Pa] -> [x4]
  [phi1_hat] -> Add1/1  "phi1_hat"
  Add1/1 -> x_bar/1
  fs_real/1 -> [f_s_real]
  [phi2_hat] -> Out1/1
  Subsystem1/1(phi2_hat_dot) -> Integrator1/1
  Integrator1/1 -> Subsystem1/8(phi2_hat), [phi2_hat]
  Square/1 -> Gain/1
  [d1_hat] -> Integrator4/1
  Integrator4/1 -> Scope1/1, Add1/2
  [f_s_real] -> Scope1/2
  Discrete Transfer Fcn1/1 -> Discrete Transfer Fcn2/1
  [phi2_hat] -> Scope2/2  "phi2_hat"

== system phdMain/Subsystem4 ==
  In1 : Inport
  Add : Sum
  Constant : Constant
  Constant1 : Constant  Value=100
  Relational Operator : RelationalOperator  OutDataTypeStr=boolean  RndMeth=Simplest  InputSameDT=off
  Saturation : Saturate  UpperLimit=100  LowerLimit=0
  Switch : Switch  Criteria=u2 ~= 0  SaturateOnIntegerOverflow=off  InputSameDT=off
  Unit Delay : UnitDelay  SampleTime=-1  HasFrameUpgradeWarning=on
  u_perc_offset : Outport
  wires:
  Constant/1 -> Add/1
  Add/1 -> Unit Delay/1, Saturation/1
  Unit Delay/1 -> Add/2
  Saturation/1 -> Relational Operator/1
  Constant1/1 -> Relational Operator/2
  Relational Operator/1 -> Switch/2
  In1/1 -> Switch/1

== system phdMain/old ==
  Bus Creator1 : BusCreator  Commented=on  Inputs=3
  Constant10 : Constant  Commented=on  Value=mean(P_supply_Pa)
  Constant4 : Constant  Commented=on  Value=mean(P_return_Pa)
  Constant6 : Constant  Commented=on  Value=mean(P_supply_Pa)
  Constant9 : Constant  Commented=on  Value=mean(P_return_Pa)
  Flow_Calc_NoLeak : Subsystem  Commented=on
  Flow_Calc_WithLeak : Subsystem  Commented=on
  From Workspace13 : FromWorkspace  Commented=on  VariableName=P_supply_Pa
  From Workspace8 : FromWorkspace  Commented=on  VariableName=P_return_Pa
  From13 : From  Commented=on  GotoTag=PA_sim_Pa
  From14 : From  Commented=on  GotoTag=PB_sim_Pa
  From15 : From  Commented=on  GotoTag=u_perc
  From23 : From  Commented=on  GotoTag=PA_sim_Pa
  From26 : From  Commented=on  GotoTag=PB_sim_Pa
  From29 : From  Commented=on  GotoTag=Q_return
  From32 : From  Commented=on  GotoTag=q_withLeaks
  From37 : From  Commented=on  GotoTag=xv
  From38 : From  Commented=on  GotoTag=PA_sim_Pa
  From39 : From  Commented=on  GotoTag=PB_sim_Pa
  From40 : From  Commented=on  GotoTag=xv
  From43 : From  Commented=on  GotoTag=xv
  Gain15 : Gain  Commented=on  Gain=50E-3/100
  Gain16 : Gain  Commented=on  Gain=m3PsToLpm
  Gain17 : Gain  Commented=on  Gain=m3PsToLpm
  Goto21 : Goto  Commented=on  GotoTag=xv
  Goto26 : Goto  Commented=on  GotoTag=q_withLeaks
  Goto27 : Goto  Commented=on  GotoTag=q_NoLeaks
  MATLAB Function2 : MATLAB Function  Commented=on  TreatAsAtomicUnit=on
  Scope14 : Scope  NumInputPorts=2
  Scope17 : Scope  Commented=on  NumInputPorts=2
  ServoValve_Dynamics : Subsystem  Commented=on
  wires:
  Constant9/1 -> MATLAB Function2/3(P_T)
  From32/1 -> Scope14/2
  Constant4/1 -> Flow_Calc_WithLeak/3(P_return)
  From26/1 -> MATLAB Function2/5(P_B)  "PB_sim_Pa"
  From Workspace13/1 -> Flow_Calc_NoLeak/2(P_supply)
  From29/1 -> Gain17/1
  Gain15/1 -> MATLAB Function2/1(xv)
  Bus Creator1/1 -> Scope14/1
  From37/1 -> Flow_Calc_WithLeak/1(xv)
  Constant10/1 -> MATLAB Function2/2(P_P)
  From Workspace8/1 -> Flow_Calc_NoLeak/3(P_return)
  MATLAB Function2/3(Q_RETURN) -> Gain16/1, Bus Creator1/3  "Q_RETURN_lpm"
  From23/1 -> MATLAB Function2/4(P_A)  "PA_sim_Pa"
  Gain16/1 -> Scope17/2  "Q_RETURN_lpm"
  MATLAB Function2/1(Q1) -> Bus Creator1/1  "q1"
  MATLAB Function2/2(Q2) -> Bus Creator1/2  "q2"
  From14/1 -> Flow_Calc_WithLeak/5(P_2)  "P_2_sim"
  From39/1 -> Flow_Calc_NoLeak/5(P_2)  "P_2_sim"
  Flow_Calc_NoLeak/1(Q) -> Goto27/1
  Flow_Calc_WithLeak/1(q_withLeaks) -> Goto26/1
  From40/1 -> Flow_Calc_NoLeak/1(xv)
  [u_sim] -> Gain15/1
  Constant6/1 -> Flow_Calc_WithLeak/2(P_supply)
  From38/1 -> Flow_Calc_NoLeak/4(P_1)  "P_1_sim"
  From13/1 -> Flow_Calc_WithLeak/4(P_1)  "P_1_sim"
  Gain17/1 -> Scope17/1  "Q_RETURN_lpmREAL"
  ServoValve_Dynamics/1(xv) -> Goto21/1  "xv"
  From15/1 -> ServoValve_Dynamics/1(u)  "u_sim"

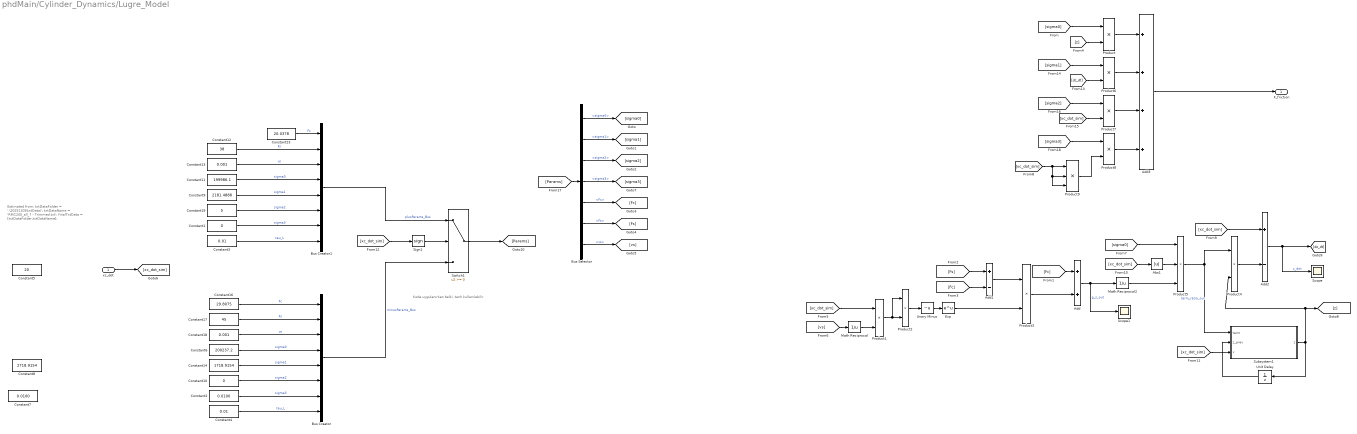
== system phdMain/Cylinder_Dynamics/Lugre_Model ==
  note: Koda uygulanırken belki, tanh kullanılabilir
  note: Estimated from:
      |
      | txtDataFolder = '.\20251105\txtData\';
      | txtDataName = 'RMC200_all_7 - Trimmed.txt';
      | finalTxtData = [txtDataFolder,txtDataName];
  xc_dot : Inport  OutDataTypeStr=double
  Abs1 : Abs  SaturateOnIntegerOverflow=off
  Add : Sum
  Add1 : Sum  Inputs=+-
  Add2 : Sum  Inputs=+-
  Add3 : Sum  Inputs=++++
  Bus Selector : BusSelector  OutputSignals=sigma0,sigma1,sigma2,sigma3,Fc,Fs,vs
  Bus Creator : BusCreator  Inputs=8
  Bus Creator1 : BusCreator  Inputs=8
  Constant1 : Constant  Value=0  OutDataTypeStr=double
  Constant10 : Constant  Value=0  OutDataTypeStr=double
  Constant11 : Constant  Value=199986.1  OutDataTypeStr=double
  Constant12 : Constant  Value=38  OutDataTypeStr=double
  Constant13 : Constant  Value=0.001  OutDataTypeStr=double
  Constant14 : Constant  Value=1718.9154  OutDataTypeStr=double
  Constant16 : Constant  Value=29.8075  OutDataTypeStr=double
  Constant17 : Constant  Value=45  OutDataTypeStr=double
  Constant18 : Constant  Value=0.001  OutDataTypeStr=double
  Constant19 : Constant  Value=5  OutDataTypeStr=double
  Constant2 : Constant  Value=0.0100  OutDataTypeStr=double
  Constant23 : Constant  Value=20.0378  OutDataTypeStr=double
  Constant3 : Constant  Value=0.01  OutDataTypeStr=double
  Constant4 : Constant  Value=0.01  OutDataTypeStr=double
  Constant5 : Constant  Value=20  OutDataTypeStr=double
  Constant6 : Constant  Value=200237.2  OutDataTypeStr=double
  Constant7 : Constant  Value=0.0100  OutDataTypeStr=double
  Constant8 : Constant  Value=2718.9154  OutDataTypeStr=double
  Constant9 : Constant  Value=2181.4888  OutDataTypeStr=double
  Exp : Math  SignedPower=on
  Math Reciprocal : Math  Operator=reciprocal  SignedPower=on
  Math Reciprocal2 : Math  Operator=reciprocal  SignedPower=on
  Product{,1..4,6..8} (8 alike) : Product
  Product5 : Product  Inputs=3
  Product9 : Product  Inputs=3
  Scope : Scope
  Scope1 : Scope
  Sign1 : Signum
  Subsystem1 : Subsystem
  Switch1 : Switch  SaturateOnIntegerOverflow=off  InputSameDT=off
  Unary Minus : UnaryMinus
  Unit Delay : UnitDelay  SampleTime=-1  HasFrameUpgradeWarning=on
  F_friction : Outport
  wires:
  Constant18/1 -> Bus Creator/3  "vs"
  Constant13/1 -> Bus Creator1/3  "vs"
  Constant12/1 -> Bus Creator1/2  "Fs"
  Constant17/1 -> Bus Creator/2  "Fs"
  Constant14/1 -> Bus Creator/5  "sigma1"
  Constant6/1 -> Bus Creator/4  "sigma0"
  Constant10/1 -> Bus Creator/6  "sigma2"
  Constant16/1 -> Bus Creator/1  "Fc"
  Constant9/1 -> Bus Creator1/5  "sigma1"
  Constant11/1 -> Bus Creator1/4  "sigma0"
  Constant19/1 -> Bus Creator1/6  "sigma2"
  Product7/1 -> Add3/3
  Product6/1 -> Add3/2
  [sigma2] -> Product7/1
  [xc_dot_sim] -> Product7/2
  [dz_dt] -> Product6/2
  [sigma1] -> Product6/1
  Product/1 -> Add3/1
  [z] -> Product/2
  [sigma0] -> Product5/1
  Abs1/1 -> Product5/2
  Add/1 -> Math Reciprocal2/1, Scope1/1  "g_s_out"
  [xc_dot_sim] -> Abs1/1
  Add1/1 -> Product3/1
  Unary Minus/1 -> Exp/1
  Product2/1 -> Unary Minus/1
  Product1/1 -> Product2/2, Product2/1
  [xc_dot_sim] -> Product1/1
  Math Reciprocal/1 -> Product1/2
  [vs] -> Math Reciprocal/1
  [Fc] -> Add1/2
  [Fs] -> Add1/1
  [Fc] -> Add/1
  [sigma0] -> Product/1
  Product3/1 -> Add/2
  [xc_dot_sim] -> Sign1/1
  Bus Creator1/1 -> Switch1/1  "plusParams_Bus"
  Bus Creator/1 -> Switch1/3  "minusParams_Bus"
  Switch1/1 -> [Params]
  [Params] -> Bus Selector/1
  Bus Selector/1 -> [sigma0]  "<sigma0>"
  Bus Selector/2 -> [sigma1]  "<sigma1>"
  Bus Selector/3 -> [sigma2]  "<sigma2>"
  Bus Selector/5 -> [Fc]  "<Fc>"
  Bus Selector/6 -> [Fs]  "<Fs>"
  Bus Selector/7 -> [vs]  "<vs>"
  Math Reciprocal2/1 -> Product5/3
  Exp/1 -> Product3/2
  Add2/1 -> Scope/1, [dz_dt]  "z_dot"
  Sign1/1 -> Switch1/2
  [xc_dot_sim] -> Add2/1
  Subsystem1/1(z) -> Product4/2, [z], Unit Delay/1
  [xc_dot_sim] -> Subsystem1/3(v)
  Unit Delay/1 -> Subsystem1/2(z_prev)
  Product5/1 -> Subsystem1/1(term), Product4/1  "term_ratio_out"
  Product4/1 -> Add2/2
  Add3/1 -> F_friction/1
  Constant1/1 -> Bus Creator1/7  "sigma3"
  Constant2/1 -> Bus Creator/7  "sigma3"
  Constant3/1 -> Bus Creator1/8  "tau_L"
  Constant4/1 -> Bus Creator/8  "tau_L"
  [sigma3] -> Product8/1
  Product8/1 -> Add3/4
  [xc_dot_sim] -> Product9/2, Product9/3, Product9/1
  Product9/1 -> Product8/2
  Bus Selector/4 -> [sigma3]  "<sigma3>"
  xc_dot/1 -> [xc_dot_sim]
  Constant23/1 -> Bus Creator1/1  "Fc"

== system phdMain/Cylinder_Dynamics/Subsystem ==
  note: Gain
  note: 7ms delay eklendi
  note: Gain
  x : Inport
  pa : Inport  Port=2
  pb : Inport  Port=3
  Add1 : Sum
  Add2 : Sum  Inputs=+++
  Add3 : Sum
  Bus Creator : BusCreator  Inputs=2
  Bus Creator1 : BusCreator  Inputs=2
  Constant : Constant  Value=0.001
  From Workspace1 : FromWorkspace  Commented=on  VariableName=F_friction
  From Workspace10 : FromWorkspace  VariableName=xc_m
  From Workspace12 : FromWorkspace  VariableName=xc_m
  From Workspace13 : FromWorkspace  VariableName=PA_Pa
  From Workspace14 : FromWorkspace  VariableName=PB_Pa
  From Workspace5 : FromWorkspace  VariableName=v_mPs
  From Workspace6 : FromWorkspace  VariableName=v_mPs
  From Workspace7 : FromWorkspace  VariableName=v_mPs
  From Workspace8 : FromWorkspace  Commented=on  VariableName=F_friction
  From Workspace9 : FromWorkspace  VariableName=a_mPs2
  Gain1 : Gain  Gain=1.5
  Gain2 : Gain  Gain=0.021
  Gain3 : Gain  Gain=0
  Gain4 : Gain  Gain=1.5
  Gain5 : Gain  Gain=0.021
  Kalman_Jerk_xPaPb : MATLAB Function  TreatAsAtomicUnit=on
  Kalman_Jerk_xa : MATLAB Function  TreatAsAtomicUnit=on
  Scope : Scope  NumInputPorts=2
  Scope1 : Scope
  Scope2 : Scope
  Subsystem : Subsystem
  Subsystem1 : Subsystem
  To Workspace : ToWorkspace  VariableName=F_Friction_Sim  SaveFormat=Timeseries  SampleTime=-1
  To Workspace1 : ToWorkspace  VariableName=V_Sim  SaveFormat=Timeseries  SampleTime=-1
  Transport Delay : TransportDelay  DelayTime=7e-3
  Unit Delay{1..4} (4 alike) : UnitDelay  SampleTime=-1  HasFrameUpgradeWarning=on
  XY Graph : Record  FileSettingsInternal="{\"entries\":[{\"content\":{\"excelSettings\":{\"content\":{},\"type\":\"Streamout.ExcelSettings\"}},\"type\":\"Streamout.FileSettingStorage\",\"uuid\":\"\"}],\"packageUris\":[\"http:\\/\\/schema.mathworks.com\\/mf0\\/streamout_blocks\\/R2020a\"],\"version\":\"1.0\"}"  Layout=[1 1]  SignalsInternal="{\"entries\":[{\"content\":{\"signals\":[{\"content\":{\"blockPath\":[],\"dimensions\":[1],\"domain\":\"\",\"hasChildren\":true,\"lineColor\":\"#77ac30\",\"port\":1,\"signalID\":26727,\"signalName\":\"Bus Creator\"},\"type\":\"RecordBlkView.Signal\",\"uuid\":\"\"},{\"content\":{\"blockPath\":[],\"dimensions\":[1],\"domain\":\"\",\"leafPath\":\"Bus Creator.signal1\",\"lineColor\":\"#fe330a\",\"parentID\":26727,\"port\":1,\"signalID\":26730,\"signalName\":\"Bus Creator.signal1\"},\"type\":\"RecordBlkView.Signal\",\"uuid\":\"\"},{\"content\":{\"blockPath\":[],\"dimensions\":[1],\"domain\":\"\",\"leafPath\":\"Bus Creator.signal2\",\"lineColor\":\"#22b573\",\"parentID\":26727,\"port\":1,\"signalID\":26733,\"signalName\":\"Bus Creator.signal2\"},\"type\":\"RecordBlkView.Signal\",\"uuid\":\"\"},{\"content\":{\"blockPath\":[],\"dimensions\":[1],\"domain\":\"\",\"hasChildren\":true,\"lineColor\":\"#139fff\",\"port\":2,\"signalID\":26736,\"signalName\":\"Bus Creator1\"},\"type\":\"RecordBlkView.Signal\",\"uuid\":\"\"},{\"content\":{\"blockPath\":[],\"dimensions\":[1],\"domain\":\"\",\"leafPath\":\"Bus Creator1.signal1\",\"lineColor\":\"#d95319\",\"parentID\":26736,\"port\":2,\"signalID\":26739,\"signalName\":\"Bus Creator1.signal1\"},\"type\":\"RecordBlkView.Signal\",\"uuid\":\"\"},{\"content\":{\"blockPath\":[],\"dimensions\":[1],\"domain\":\"\",\"leafPath\":\"Bus Creator1.signal2\",\"lineColor\":\"#edb120\",\"parentID\":26736,\"port\":2,\"signalID\":26742,\"signalName\":\"Bus Creator1.signal2\"},\"type\":\"RecordBlkView.Signal\",\"uuid\":\"\"}]},\"type\":\"RecordBlkView.InputSignals\",\"uuid\":\"\"}],\"packageUris\":[\"http:\\/\\/schema.mathworks.com\\/mf0\\/streamout_blocks\\/R2020a\"],\"version\":\"1.0\"}"  VisualizationBindings="{\"xyplotplugin\":{\"info\":[{\"series\":[],\"subplotID\":1}]}}"  CompatibilityTag=XY
  FRIC : Outport
  FRIC1 : Outport  Port=2
  wires:
  Unit Delay2/1 -> Bus Creator1/2
  From Workspace9/1 -> Kalman_Jerk_xa/2(acc_meas)
  Constant/1 -> Kalman_Jerk_xa/3(dt)
  From Workspace12/1 -> Scope2/1, Kalman_Jerk_xPaPb/1(pos_meas)
  From Workspace7/1 -> Unit Delay3/1
  Unit Delay3/1 -> Bus Creator1/1
  From Workspace13/1 -> Kalman_Jerk_xPaPb/2(PA)
  Add3/1 -> Transport Delay/1
  Bus Creator1/1 -> XY Graph/2
  From Workspace10/1 -> Kalman_Jerk_xa/1(pos_meas)
  From Workspace5/1 -> Unit Delay1/1
  Bus Creator/1 -> XY Graph/1
  From Workspace14/1 -> Kalman_Jerk_xPaPb/3(PB)
  Kalman_Jerk_xPaPb/1(j_est) -> Gain2/1
  From Workspace8/1 -> Unit Delay2/1
  Kalman_Jerk_xPaPb/2(a_est) -> Gain1/1
  From Workspace6/1 -> To Workspace1/1
  Unit Delay1/1 -> Bus Creator/1
  Kalman_Jerk_xPaPb/3(v_est) -> Scope1/1, Subsystem/1(v_est)
  From Workspace1/1 -> Unit Delay4/1
  Unit Delay4/1 -> Scope/1
  Transport Delay/1 -> Scope/2, FRIC/1, Bus Creator/2, To Workspace/1
  Subsystem/1(F_statik) -> Add1/2
  Gain1/1 -> Add1/1
  Gain2/1 -> Gain3/1
  Add1/1 -> Add3/2
  Gain3/1 -> Add3/1
  Kalman_Jerk_xa/2(a_est) -> Gain4/1
  Kalman_Jerk_xa/1(v_est) -> Subsystem1/1(v_est)
  Subsystem1/1(F_statik) -> Add2/1
  Gain4/1 -> Add2/2
  Add2/1 -> FRIC1/1
  Kalman_Jerk_xa/3(j_est) -> Gain5/1
  Gain5/1 -> Add2/3

== system phdMain/Cylinder_Dynamics/Subsystem1 ==
  Constant2 : Constant  Value=-0.09580
  Constant5 : Constant  Value=0.09580
  Constant6 : Constant  Value=1e6
  Constant7 : Constant  Value=2e-3
  MATLAB Function1 : MATLAB Function  TreatAsAtomicUnit=on
  F_end : Outport
  wires:
  Constant7/1 -> MATLAB Function1/6(v_lock)
  [xc_sim] -> MATLAB Function1/1(x)
  [xc_dot_sim] -> MATLAB Function1/2(x_dot)
  Constant6/1 -> MATLAB Function1/5(k_end)
  Constant2/1 -> MATLAB Function1/3(xmin)
  Constant5/1 -> MATLAB Function1/4(xmax)
  MATLAB Function1/1(F_end) -> F_end/1
